simulink model "Motor5_Avellaneda"  (R2023b)
settings: Solver=FixedStepAuto  StartTime=0.0  StopTime=0.12  FixedStep=1e-4  RelTol=1e-3
undefined symbols (not defined in the file or in its folder): C, f, F, G, K, KI, L
settings Model: Creator=Usuario  LastModifiedBy=Usuario

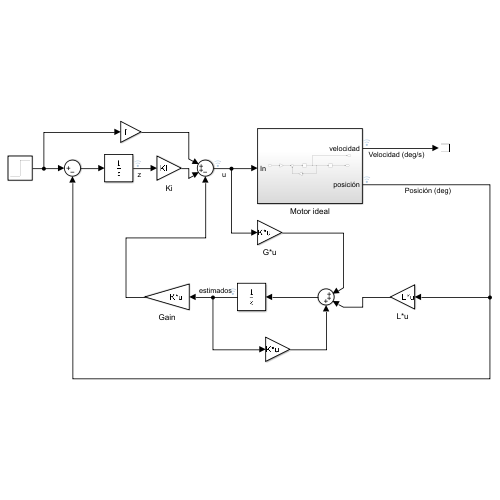
[thumbnail: Simulink's stored preview of the top-level diagram]
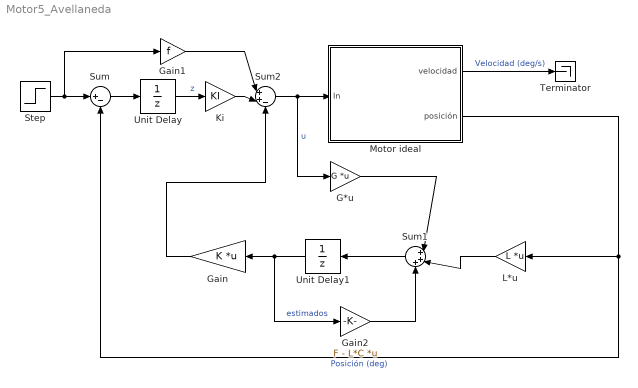
== system Motor5_Avellaneda ==
  G*u : Gain  Gain=G  Multiplication=Matrix(K*u)
  Gain : Gain  Gain=K  Multiplication=Matrix(K*u)
  Gain1 : Gain  Gain=f
  Gain2 : Gain  Gain=F - L*C  Multiplication=Matrix(K*u)
  Ki : Gain  Gain=KI
  L*u : Gain  Gain=L  Multiplication=Matrix(K*u)
  Motor ideal : Subsystem
  Step : Step  Time=0  After=540  SampleTime=0
  Sum : Sum  Inputs=|+-
  Sum1 : Sum  Inputs=|+++
  Sum2 : Sum  Inputs=|++-
  Terminator : Terminator
  Unit Delay : UnitDelay  SampleTime=0.0001  HasFrameUpgradeWarning=on
  Unit Delay1 : UnitDelay  SampleTime=0.0001  HasFrameUpgradeWarning=on
  wires:
  Motor ideal/1(velocidad) -> Terminator/1  "Velocidad (deg/s)"
  Motor ideal/2(posición) -> Sum/2, L*u/1  "Posición (deg)"
  G*u/1 -> Sum1/1
  L*u/1 -> Sum1/2
  Sum1/1 -> Unit Delay1/1
  Unit Delay1/1 -> Gain2/1, Gain/1  "estimados"
  Gain2/1 -> Sum1/3
  Step/1 -> Gain1/1, Sum/1
  Sum/1 -> Unit Delay/1
  Unit Delay/1 -> Ki/1  "z"
  Sum2/1 -> G*u/1, Motor ideal/1(In)  "u"
  Ki/1 -> Sum2/2
  Gain1/1 -> Sum2/1
  Gain/1 -> Sum2/3

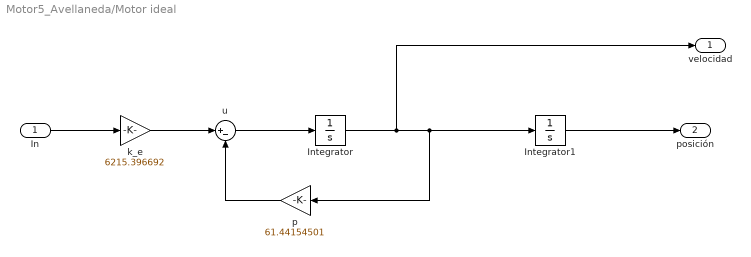
== system Motor5_Avellaneda/Motor ideal ==
  In : Inport
  Integrator : Integrator  InitialCondition=1
  Integrator1 : Integrator  InitialCondition=2
  k_e : Gain  Gain=6215.396692
  p : Gain  Gain=61.44154501
  u : Sum  Inputs=|+-
  velocidad : Outport
  posición : Outport  Port=2
  wires:
  Integrator/1 -> Integrator1/1, p/1, velocidad/1
  u/1 -> Integrator/1
  p/1 -> u/2
  k_e/1 -> u/1
  Integrator1/1 -> posición/1
  In/1 -> k_e/1
